simulink model "testcchannel"  (Simulink 7.1)
settings: Solver=ode45  StartTime=0.0  StopTime=0.0  RelTol=1e-3
undefined symbols (not defined in the file): IScale
libraries: SaliencyLib x11
settings Model: Creator=bruce  LastModifiedBy=bruce

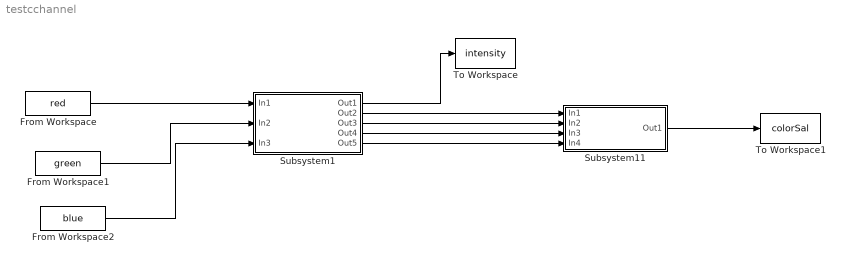
== system testcchannel ==
  From Workspace : FromWorkspace  VariableName=red  SampleTime=0
  From Workspace1 : FromWorkspace  VariableName=green  SampleTime=0
  From Workspace2 : FromWorkspace  VariableName=blue  SampleTime=0
  Subsystem1 : Subsystem
      mask Display:
      | disp('COLOR\nMAPPING')
      | port_label('input',1,'r')
      | port_label('input',2','g')
      | port_label('input',3,'b')
      | port_label('output',1,'I')
      | port_label('output',2,'R')
      | port_label('output',3,'G')
      | port_label('output',4','B')
      | port_label('output',5,'Y')
  Subsystem11 : Subsystem
      mask Display: disp('COLOR CHANNEL')
  To Workspace : ToWorkspace  VariableName=intensity  SampleTime=-1  SaveFormat=Structure
  To Workspace1 : ToWorkspace  VariableName=colorSal  SampleTime=-1  SaveFormat=Structure
  wires:
  From Workspace/1 -> Subsystem1/1(In1)
  Subsystem1/1(Out1) -> To Workspace/1
  From Workspace1/1 -> Subsystem1/2(In2)
  From Workspace2/1 -> Subsystem1/3(In3)
  Subsystem1/2(Out2) -> Subsystem11/1(In1)
  Subsystem1/3(Out3) -> Subsystem11/2(In2)
  Subsystem1/4(Out4) -> Subsystem11/3(In3)
  Subsystem1/5(Out5) -> Subsystem11/4(In4)
  Subsystem11/1(Out1) -> To Workspace1/1

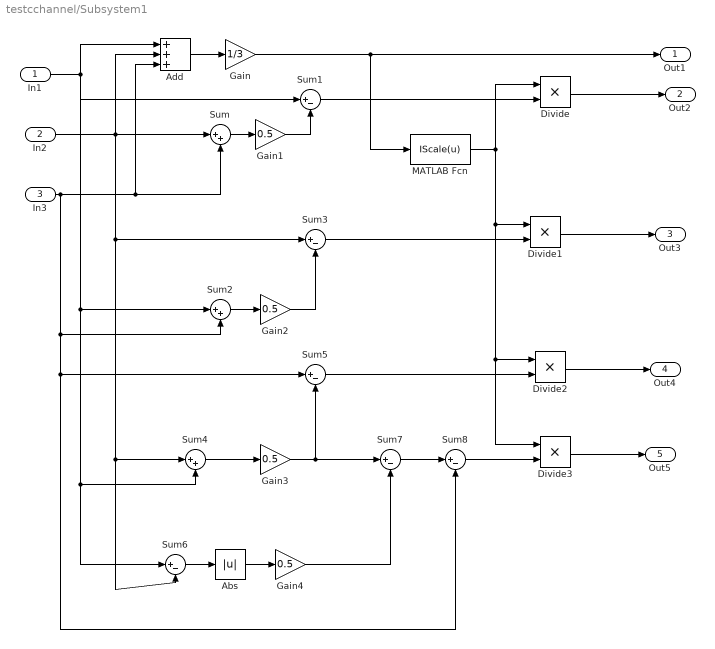
== system testcchannel/Subsystem1 ==
  In1 : Inport  OutDataType=sfix(16)  OutScaling=2^0
  In2 : Inport  Port=2  OutDataType=sfix(16)  OutScaling=2^0
  In3 : Inport  Port=3  OutDataType=sfix(16)  OutScaling=2^0
  Abs : Abs  OutDataType=sfix(16)  OutScaling=2^0
  Add : Sum  Inputs=+++  OutDataType=sfix(16)  OutScaling=2^-10
  Divide{,1..3} (4 alike) : Product  Inputs=**  OutDataType=sfix(16)  OutScaling=2^-10
  Gain : Gain  Gain=1/3  ParameterDataType=sfix(16)  ParameterScaling=2^0  OutDataType=sfix(16)  OutScaling=2^0
  Gain{1..4} (4 alike) : Gain  Gain=0.5  ParameterDataType=sfix(16)  ParameterScaling=2^0  OutDataType=sfix(16)  OutScaling=2^0
  MATLAB Fcn : MATLABFcn  MATLABFcn=IScale(u)  Output1D=off
  Sum : Sum  Inputs=|++  OutDataType=sfix(16)  OutScaling=2^0
  Sum{1,3,5..8} (6 alike) : Sum  Inputs=|+-  OutDataType=sfix(16)  OutScaling=2^0
  Sum2 : Sum  Inputs=|++  OutDataType=sfix(16)  OutScaling=2^0
  Sum4 : Sum  Inputs=|++  OutDataType=sfix(16)  OutScaling=2^0
  Out1 : Outport  OutDataType=sfix(16)  OutScaling=2^0
  Out2 : Outport  Port=2  OutDataType=sfix(16)  OutScaling=2^0
  Out3 : Outport  Port=3  OutDataType=sfix(16)  OutScaling=2^0
  Out4 : Outport  Port=4  OutDataType=sfix(16)  OutScaling=2^0
  Out5 : Outport  Port=5  OutDataType=sfix(16)  OutScaling=2^0
  wires:
  MATLAB Fcn/1 -> Divide3/1, Divide2/1, Divide1/1, Divide/1
  Divide3/1 -> Out5/1
  Sum8/1 -> Divide3/2
  Sum7/1 -> Sum8/1
  Gain4/1 -> Sum7/2
  Abs/1 -> Gain4/1
  Sum6/1 -> Abs/1
  Divide2/1 -> Out4/1
  Divide1/1 -> Out3/1
  Sum5/1 -> Divide2/2
  Sum3/1 -> Divide1/2
  Divide/1 -> Out2/1
  Sum1/1 -> Divide/2
  Sum4/1 -> Gain3/1
  Gain3/1 -> Sum7/1, Sum5/2
  Gain2/1 -> Sum3/2
  Sum2/1 -> Gain2/1
  Gain1/1 -> Sum1/2
  Sum/1 -> Gain1/1
  Add/1 -> Gain/1
  Gain/1 -> MATLAB Fcn/1, Out1/1
  In3/1 -> Sum8/2, Sum5/1, Sum2/2, Sum/2, Add/3
  In2/1 -> Sum6/2, Sum4/1, Sum3/1, Sum/1, Add/2
  In1/1 -> Sum6/1, Sum4/2, Sum2/1, Sum1/1, Add/1

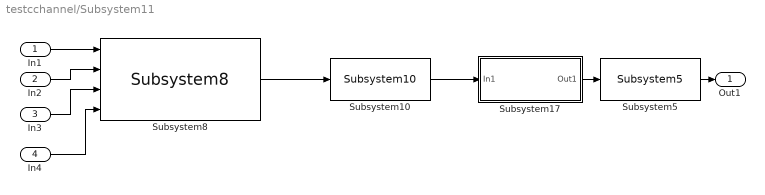
== system testcchannel/Subsystem11 ==
  In1 : Inport  OutDataType=sfix(16)  OutScaling=2^0
  In2 : Inport  Port=2  OutDataType=sfix(16)  OutScaling=2^0
  In3 : Inport  Port=3  OutDataType=sfix(16)  OutScaling=2^0
  In4 : Inport  Port=4  OutDataType=sfix(16)  OutScaling=2^0
  Subsystem10 : SaliencyLib/Subsystem10  SystemSampleTime=-1
  Subsystem17 : Subsystem  AncestorBlock=SaliencyLib/Subsystem17  mask{l2r=83, l2c=125, l3r=42, l3c=63}
      mask prompts: l2r "L2 rows:"; l2c "L2 cols:"; l3r "L3 rows:"; l3c "L3 cols:"
      mask Display: disp('X-SCALE\nCOMBINE')
  Subsystem5 : SaliencyLib/Subsystem5  SystemSampleTime=-1
  Subsystem8 : SaliencyLib/Subsystem8  SystemSampleTime=-1  br=332  bc=500
  Out1 : Outport  OutDataType=sfix(16)  OutScaling=2^0
  wires:
  In4/1 -> Subsystem8/4
  In3/1 -> Subsystem8/3
  In2/1 -> Subsystem8/2
  Subsystem5/1 -> Out1/1
  Subsystem17/1(Out1) -> Subsystem5/1
  Subsystem10/1 -> Subsystem17/1(In1)
  Subsystem8/1 -> Subsystem10/1
  In1/1 -> Subsystem8/1

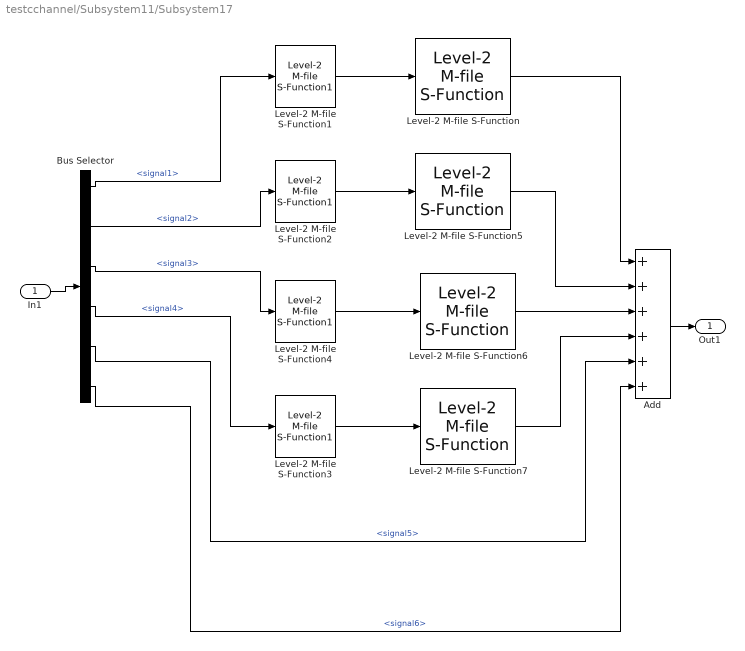
== system testcchannel/Subsystem11/Subsystem17 ==
  In1 : Inport  OutDataType=sfix(16)  OutScaling=2^0
  Add : Sum  Inputs=++++++  OutDataType=sfix(16)  OutScaling=2^-10
  Bus Selector : BusSelector  OutputSignals=signal1,signal2,signal3,signal4,signal5,signal6
  Level-2 M-file S-Function : SaliencyLib/Level-2 M-file S-Function  br=l2r  bc=l2c  pl=2
  Level-2 M-file S-Function1 : SaliencyLib/Level-2 M-file S-Function1  sr=l2r  sc=l2c  sl=2
  Level-2 M-file S-Function2 : SaliencyLib/Level-2 M-file S-Function1  sr=l2r  sc=l2c  sl=2
  Level-2 M-file S-Function3 : SaliencyLib/Level-2 M-file S-Function1  sr=l3r  sc=l3c  sl=1
  Level-2 M-file S-Function4 : SaliencyLib/Level-2 M-file S-Function1  sr=l3r  sc=l3c  sl=1
  Level-2 M-file S-Function5 : SaliencyLib/Level-2 M-file S-Function  br=l2r  bc=l2c  pl=2
  Level-2 M-file S-Function6 : SaliencyLib/Level-2 M-file S-Function  br=l3r  bc=l3c  pl=1
  Level-2 M-file S-Function7 : SaliencyLib/Level-2 M-file S-Function  br=l3r  bc=l3c  pl=1
  Out1 : Outport  OutDataType=sfix(16)  OutScaling=2^0
  wires:
  Level-2 M-file S-Function1/1 -> Level-2 M-file S-Function/1
  Level-2 M-file S-Function2/1 -> Level-2 M-file S-Function5/1
  Level-2 M-file S-Function4/1 -> Level-2 M-file S-Function6/1
  Level-2 M-file S-Function3/1 -> Level-2 M-file S-Function7/1
  Level-2 M-file S-Function/1 -> Add/1
  Level-2 M-file S-Function5/1 -> Add/2
  Level-2 M-file S-Function6/1 -> Add/3
  Level-2 M-file S-Function7/1 -> Add/4
  Add/1 -> Out1/1
  Bus Selector/1 -> Level-2 M-file S-Function1/1  "<signal1>"
  Bus Selector/2 -> Level-2 M-file S-Function2/1  "<signal2>"
  Bus Selector/3 -> Level-2 M-file S-Function4/1  "<signal3>"
  Bus Selector/4 -> Level-2 M-file S-Function3/1  "<signal4>"
  Bus Selector/5 -> Add/5  "<signal5>"
  Bus Selector/6 -> Add/6  "<signal6>"
  In1/1 -> Bus Selector/1
